simulink subsystem "damping_estimation"  (R2021b)
settings: Solver=VariableStepAuto  StartTime=0.0  StopTime=10.0  RelTol=1e-3
values from neighbouring files (symbols this model uses):
  b_c = 0    [scene_parameters.m]
  b_lb = -0.5    [scene_parameters.m]
  b_ub = 1    [scene_parameters.m]
  k_n = -log((1+sensitivity_measure)/(1-sensitivity_measure))/pd_x_pdd_min    [scene_parameters.m]
  k_p = -log((1-sensitivity_measure)/(1+sensitivity_measure))/pd_x_pdd_max    [scene_parameters.m]
settings Model: Creator=jensh  LastModifiedBy=jensh

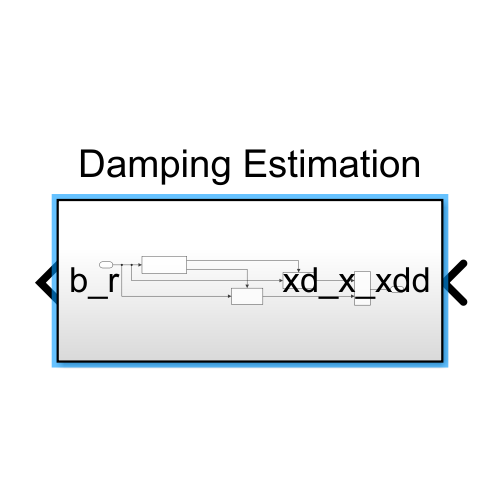
[thumbnail: Simulink's stored preview of the top-level diagram]
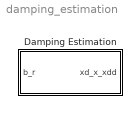
== system damping_estimation ==
  Damping Estimation : Subsystem

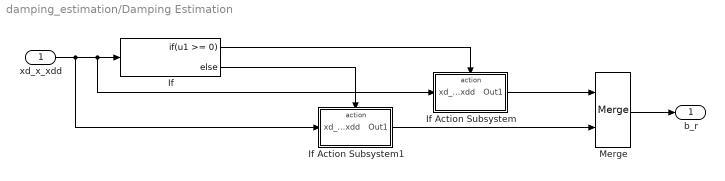
== system damping_estimation/Damping Estimation ==
  xd_x_xdd : Inport
  If : If  IfExpression=u1 >= 0
  If Action Subsystem : Subsystem  TreatAsAtomicUnit=on
  If Action Subsystem1 : Subsystem  TreatAsAtomicUnit=on
  Merge : Merge
  b_r : Outport
  wires:
  xd_x_xdd/1 -> If Action Subsystem1/1(xd_x_xdd), If Action Subsystem/1(xd_x_xdd), If/1
  If Action Subsystem1/1(Out1) -> Merge/2
  If Action Subsystem/1(Out1) -> Merge/1
  If/1 -> If Action Subsystem/Action
  If/2 -> If Action Subsystem1/Action
  Merge/1 -> b_r/1

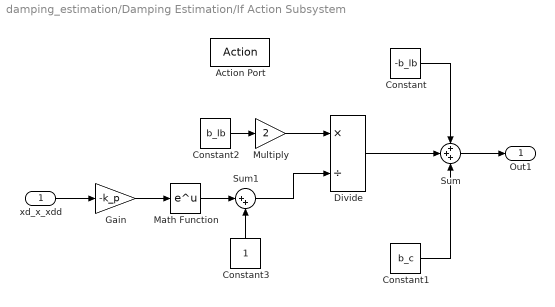
== system damping_estimation/Damping Estimation/If Action Subsystem ==
  xd_x_xdd : Inport
  Action Port : ActionPort
  Constant : Constant  Value=-b_lb
  Constant1 : Constant  Value=b_c
  Constant2 : Constant  Value=b_lb
  Constant3 : Constant
  Divide : Product  Inputs=*/
  Gain : Gain  Gain=-k_p
  Math Function : Math  SaturateOnIntegerOverflow=on
  Multiply : Gain  Gain=2
  Sum : Sum  Inputs=+++
  Sum1 : Sum  Inputs=|++
  Out1 : Outport
  wires:
  Sum/1 -> Out1/1
  Constant/1 -> Sum/1
  Constant1/1 -> Sum/3
  Divide/1 -> Sum/2
  Multiply/1 -> Divide/1
  Constant2/1 -> Multiply/1
  Sum1/1 -> Divide/2
  Constant3/1 -> Sum1/2
  Math Function/1 -> Sum1/1
  xd_x_xdd/1 -> Gain/1
  Gain/1 -> Math Function/1

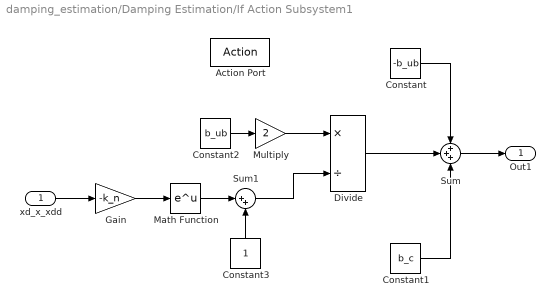
== system damping_estimation/Damping Estimation/If Action Subsystem1 ==
  xd_x_xdd : Inport
  Action Port : ActionPort
  Constant : Constant  Value=-b_ub
  Constant1 : Constant  Value=b_c
  Constant2 : Constant  Value=b_ub
  Constant3 : Constant
  Divide : Product  Inputs=*/
  Gain : Gain  Gain=-k_n
  Math Function : Math  SaturateOnIntegerOverflow=on
  Multiply : Gain  Gain=2
  Sum : Sum  Inputs=+++
  Sum1 : Sum  Inputs=|++
  Out1 : Outport
  wires:
  Sum/1 -> Out1/1
  Constant/1 -> Sum/1
  Constant1/1 -> Sum/3
  Divide/1 -> Sum/2
  Multiply/1 -> Divide/1
  Constant2/1 -> Multiply/1
  Sum1/1 -> Divide/2
  Constant3/1 -> Sum1/2
  Math Function/1 -> Sum1/1
  xd_x_xdd/1 -> Gain/1
  Gain/1 -> Math Function/1
